simulink model "PubIfControlLATC_MDL"  (R2020b)
settings: configuration reference "DspaceConfig" (kept outside this file)
PostLoadFcn:
  | if any(exist('dsrtsu_mdlpostloadfcn', 'file') ~= 0), dsrtsu_mdlpostloadfcn('Execute', bdroot); end
InitFcn:
  | , if any(exist('rtifpga_mdlclblib', 'file') ~= 0), rtifpga_mdlclblib('Init', bdroot); end,
  | , if any(exist('dsmpb_private', 'file') ~= 0), dsmpb_private('dsmpb_mdlclblib', 'Init', bdroot); end,
undefined symbols (not defined in the file or in its folder): EPS_DrvInpTrqVal_HighReslolution, EPS_FailSts, EPS_LKAAngDlvdSts, EPS_LKATorqOvrlDlvd, EPS_LKATorqOvrlDlvdVld, EPS_LKATrqOvlDlvdSts, SteerWheelAng, SteerWheelAngSign, SteerWheelSpd, SteerWheelSpdSign
PreSaveFcn:
  | , if any(exist('dsmpb_private', 'file') ~= 0), dsmpb_private('dsmpb_mdlclblib', 'PreSave', bdroot); end,
CloseFcn:
  | , if any(exist('dsmpb_private', 'file') ~= 0), dsmpb_private('dsmpb_mdlclblib', 'Close', bdroot); end,
settings Model: DataDictionary=HWA_DDs.sldd  RTICANMMDATA=struct('GeneralSetupData',struct('modelroot','D:\10_HWA_Project\Git_ADAS_Store\Adas\LATC','generalsettings',struct('filesettings',struct('destfolder',struct('Name','RTICANMM_FILES','Check',1),'buildfolder',struct('Name','.','Check',1),'AbsDestfolder',struct('Name','D:\10_HWA_Project\Git_ADAS_Store\Adas\LATC\RTICANMM_FILES'),'AbsBuildfolder',struct('Name','D:\10_HWA_Project\Git_ADAS_Store\Adas\LATC'))),'options',struct('addpaths',1,'rmpaths',1,'addtrcexclusion',false,'cannavigator',struct('checkmonitoring',0),'show_usrtrc',0,'use_usrtrc',0),'advanced',struct('options',ones(1,100)),'MPSetup',{{}},'RTI',struct('Type','DSRT','Ver','4.4','Date','02-Nov-2020'),'modelname','PubIfControlLATC_MDL','block','PubIfControlLATC_MDL'))  DSRTSU_INTERNAL_RTIFPGA=170  DSMPB_ID_DATA={}  OrderedModelArguments=off  Creator=GW00180895  LastModifiedBy=GW00201118
settings ConfigSetRef: SourceName=DspaceConfig

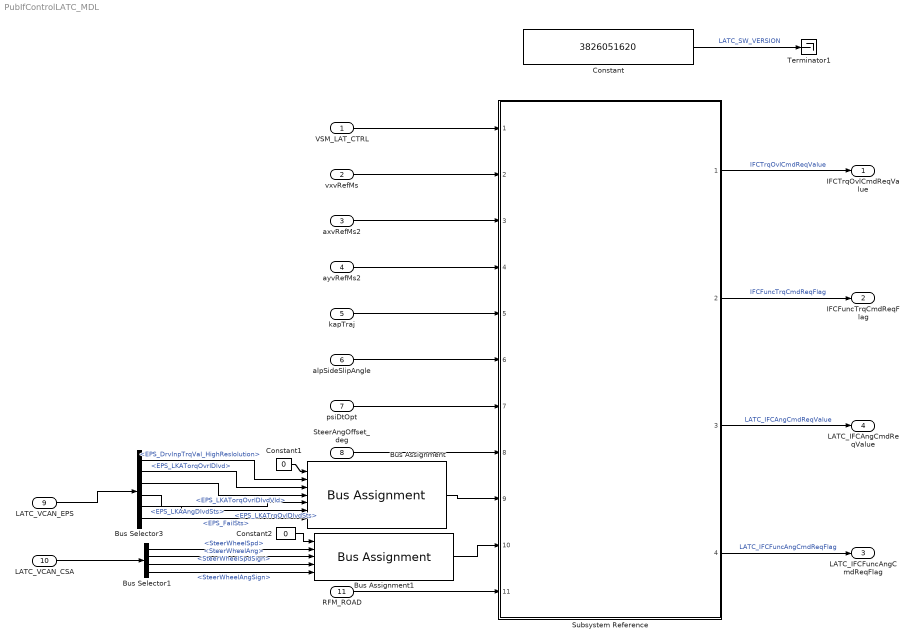
== system PubIfControlLATC_MDL ==
  VSM_LAT_CTRL : Inport  OutDataTypeStr=Bus: VSM_LAT_CTRL_BUS  PortDimensions=1  Interpolate=off  BusOutputAsStruct=on
  vxvRefMs : Inport  Port=2  OutDataTypeStr=single  PortDimensions=1  Interpolate=off  BusOutputAsStruct=on
  axvRefMs2 : Inport  Port=3  OutDataTypeStr=single  PortDimensions=1  Interpolate=off  BusOutputAsStruct=on
  ayvRefMs2 : Inport  Port=4  OutDataTypeStr=single  PortDimensions=1  Interpolate=off  BusOutputAsStruct=on
  kapTraj : Inport  Port=5  OutDataTypeStr=single  PortDimensions=1  Interpolate=off  BusOutputAsStruct=on
  alpSideSlipAngle : Inport  Port=6  OutDataTypeStr=single  PortDimensions=1  Interpolate=off  BusOutputAsStruct=on
  psiDtOpt : Inport  Port=7  OutDataTypeStr=single  PortDimensions=1  Interpolate=off  BusOutputAsStruct=on
  SteerAngOffset_deg : Inport  Port=8  OutDataTypeStr=single  PortDimensions=1  Interpolate=off  BusOutputAsStruct=on
  LATC_VCAN_EPS : Inport  Port=9  OutDataTypeStr=Bus: LATC_VCAN_EPS_BUS  PortDimensions=1  Interpolate=off  BusOutputAsStruct=on
  LATC_VCAN_CSA : Inport  Port=10  OutDataTypeStr=Bus: LATC_VCAN_CSA_BUS  PortDimensions=1  Interpolate=off  BusOutputAsStruct=on
  RFM_ROAD : Inport  Port=11  OutDataTypeStr=Bus: RFM_ROAD_BUS  PortDimensions=1  Interpolate=off  BusOutputAsStruct=on
  Bus Assignment : BusAssignment  AssignedSignals=EPS_DrvInpTrqVal_HighReslolution,EPS_LKATorqOvrlDlvd,EPS_LKATorqOvrlDlvdVld,EPS_LKAAngDlvdSts,EPS_LKATrqOvlDlvdSts,EPS_FailSts
  Bus Assignment1 : BusAssignment  AssignedSignals=SteerWheelSpd,SteerWheelAng,SteerWheelSpdSign,SteerWheelAngSign
  Bus Selector1 : BusSelector  OutputSignals=SteerWheelSpd,SteerWheelAng,SteerWheelSpdSign,SteerWheelAngSign
  Bus Selector3 : BusSelector  OutputSignals=EPS_DrvInpTrqVal_HighReslolution,EPS_LKATorqOvrlDlvd,EPS_LKATorqOvrlDlvdVld,EPS_LKAAngDlvdSts,EPS_LKATrqOvlDlvdSts,EPS_FailSts
  Constant : Constant  Value=3826051620  OutDataTypeStr=uint32
  Constant1 : Constant  Value=0  OutDataTypeStr=Bus: VCAN_EPS_MSG_BUS
  Constant2 : Constant  Value=0  OutDataTypeStr=Bus: VCAN_CSA_MSG_BUS
  Subsystem Reference : Subsystem  ReferencedSubsystem=PvtSubSys_LATC
  Terminator1 : Terminator
  IFCTrqOvlCmdReqValue : Outport  OutDataTypeStr=single  PortDimensions=1  BusOutputAsStruct=on
  IFCFuncTrqCmdReqFlag : Outport  Port=2  OutDataTypeStr=uint8  PortDimensions=1  BusOutputAsStruct=on
  LATC_IFCFuncAngCmdReqFlag : Outport  Port=3  OutDataTypeStr=uint8  PortDimensions=1  BusOutputAsStruct=on
  LATC_IFCAngCmdReqValue : Outport  Port=4  OutDataTypeStr=single  PortDimensions=1  BusOutputAsStruct=on
  wires:
  Bus Selector1/4 -> Bus Assignment1/5  "<SteerWheelAngSign>"
  psiDtOpt/1 -> Subsystem Reference/7
  axvRefMs2/1 -> Subsystem Reference/3
  Subsystem Reference/3 -> LATC_IFCAngCmdReqValue/1  "LATC_IFCAngCmdReqValue"
  SteerAngOffset_deg/1 -> Subsystem Reference/8
  Bus Selector1/2 -> Bus Assignment1/3  "<SteerWheelAng>"
  Constant/1 -> Terminator1/1  "LATC_SW_VERSION"
  Constant2/1 -> Bus Assignment1/1
  VSM_LAT_CTRL/1 -> Subsystem Reference/1
  alpSideSlipAngle/1 -> Subsystem Reference/6
  Bus Selector1/3 -> Bus Assignment1/4  "<SteerWheelSpdSign>"
  vxvRefMs/1 -> Subsystem Reference/2
  Subsystem Reference/2 -> IFCFuncTrqCmdReqFlag/1  "IFCFuncTrqCmdReqFlag"
  Bus Assignment1/1 -> Subsystem Reference/10
  kapTraj/1 -> Subsystem Reference/5
  Constant1/1 -> Bus Assignment/1
  LATC_VCAN_CSA/1 -> Bus Selector1/1
  ayvRefMs2/1 -> Subsystem Reference/4
  RFM_ROAD/1 -> Subsystem Reference/11
  Bus Assignment/1 -> Subsystem Reference/9
  LATC_VCAN_EPS/1 -> Bus Selector3/1
  Subsystem Reference/1 -> IFCTrqOvlCmdReqValue/1  "IFCTrqOvlCmdReqValue"
  Subsystem Reference/4 -> LATC_IFCFuncAngCmdReqFlag/1  "LATC_IFCFuncAngCmdReqFlag"
  Bus Selector1/1 -> Bus Assignment1/2  "<SteerWheelSpd>"
  Bus Selector3/1 -> Bus Assignment/2  "<EPS_DrvInpTrqVal_HighReslolution>"
  Bus Selector3/2 -> Bus Assignment/3  "<EPS_LKATorqOvrlDlvd>"
  Bus Selector3/3 -> Bus Assignment/4  "<EPS_LKATorqOvrlDlvdVld>"
  Bus Selector3/4 -> Bus Assignment/5  "<EPS_LKAAngDlvdSts>"
  Bus Selector3/5 -> Bus Assignment/6  "<EPS_LKATrqOvlDlvdSts>"
  Bus Selector3/6 -> Bus Assignment/7  "<EPS_FailSts>"
